simulink model "LLC_2converter"  (R2024a)
settings: Solver=ode1  StartTime=0.0  StopTime=0.05  FixedStep=1e-7  RelTol=1e-3
libraries: spsSeriesRLCBranchLib x6, spsCurrentMeasurementLib x4, spsDiodeLib x4, spsMosfetLib x2, spsVoltageMeasurementLib x2, spsLinearTransformerLib x1, spsPVArrayLib x1, sps_lib x1
settings Model: Creator=HP  LastModifiedBy=sampurnanand

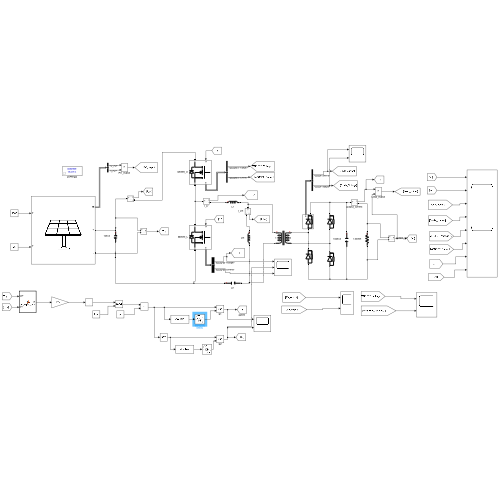
[thumbnail: Simulink's stored preview of the top-level diagram]
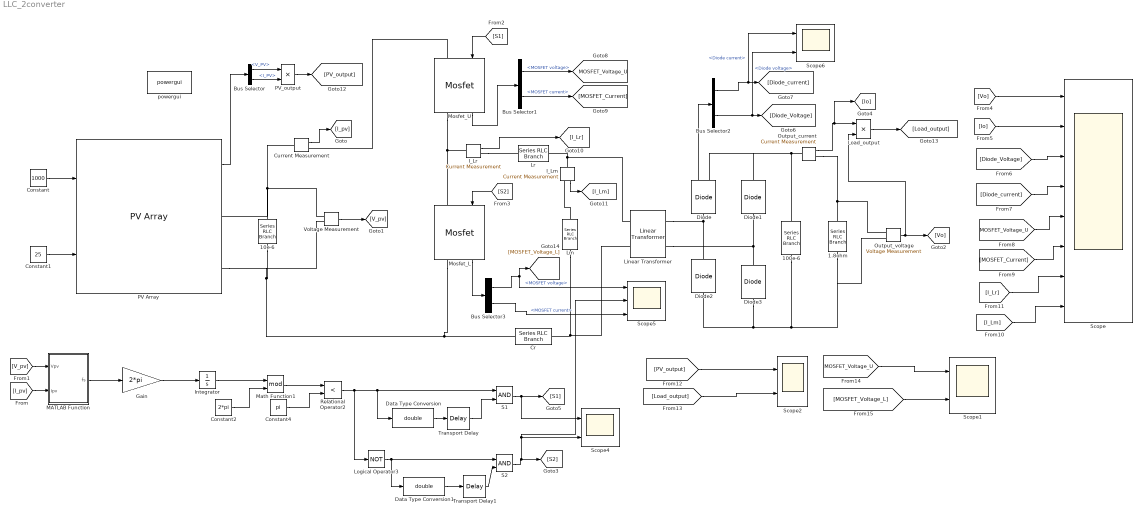
== system LLC_2converter ==
  1.8ohm : spsSeriesRLCBranchLib/Series RLC Branch  LConnTagsString=__new0  RConnTagsString=__new0  BranchType=R  Resistance=1.8  Inductance=1e-3  SetiL0=off  InitialCurrent=0  Capacitance=1e-6  Setx0=off  InitialVoltage=0  Measurements=None
  100e-6 : spsSeriesRLCBranchLib/Series RLC Branch  LConnTagsString=__new0  RConnTagsString=__new0  BranchType=C  Resistance=1  Inductance=1e-3  SetiL0=off  InitialCurrent=0  Capacitance=470e-6  Setx0=off  InitialVoltage=0  Measurements=None
  10e-6 : spsSeriesRLCBranchLib/Series RLC Branch  LConnTagsString=__new0  RConnTagsString=__new0  BranchType=C  Resistance=1  Inductance=1e-3  SetiL0=off  InitialCurrent=0  Capacitance=10e-5  Setx0=off  InitialVoltage=0  Measurements=None
  Bus Selector : BusSelector  OutputSignals=V_PV,I_PV
  Bus Selector1 : BusSelector  OutputSignals=MOSFET voltage,MOSFET current
  Bus Selector2 : BusSelector  OutputSignals=Diode current,Diode voltage
  Bus Selector3 : BusSelector  OutputSignals=MOSFET voltage,MOSFET current
  Constant : Constant  Value=1000
  Constant1 : Constant  Value=25
  Constant2 : Constant  Value=2*pi
  Constant4 : Constant  Value=pi
  Cr : spsSeriesRLCBranchLib/Series RLC Branch  LConnTagsString=__new0  RConnTagsString=__new0  BranchType=C  Resistance=1  Inductance=1e-3  SetiL0=off  InitialCurrent=0  Capacitance=3272e-9  Setx0=off  InitialVoltage=0  Measurements=None
  Current Measurement : spsCurrentMeasurementLib/Current Measurement  PhasorSimulation=off  OutputType=Complex  PSBequivalent=0
  Data Type Conversion : DataTypeConversion  OutDataTypeStr=double  SaturateOnIntegerOverflow=off  RndMeth=Floor
  Data Type Conversion1 : DataTypeConversion  OutDataTypeStr=double  SaturateOnIntegerOverflow=off  RndMeth=Floor
  Diode : spsDiodeLib/Diode  Ron=0.001  Lon=0  Vf=0.8  IC=0  UseSnubber=0  Rs=500  Cs=250e-9  Measurements=on
  Diode1 : spsDiodeLib/Diode  Ron=0.001  Lon=0  Vf=0.8  IC=0  UseSnubber=0  Rs=500  Cs=250e-9  Measurements=off
  Diode2 : spsDiodeLib/Diode  Ron=0.001  Lon=0  Vf=0.8  IC=0  UseSnubber=0  Rs=500  Cs=250e-9  Measurements=off
  Diode3 : spsDiodeLib/Diode  Ron=0.001  Lon=0  Vf=0.8  IC=0  UseSnubber=0  Rs=500  Cs=250e-9  Measurements=off
  Gain : Gain  Gain=2*pi
  I_Lm : spsCurrentMeasurementLib/Current Measurement  PhasorSimulation=off  OutputType=Complex  PSBequivalent=0
  I_Lr : spsCurrentMeasurementLib/Current Measurement  PhasorSimulation=off  OutputType=Complex  PSBequivalent=0
  Integrator : Integrator
  Linear Transformer : spsLinearTransformerLib/Linear Transformer  UNITS=SI  NominalPower=[2000 100e3]  winding1=[1 0 0]  winding2=[1 0 0]  ThreeWindings=off  winding3=[3.15e+05 0.7938 0.10107]  RmLm=[500 0]  Measurements=None  DataType=on
  Lm : spsSeriesRLCBranchLib/Series RLC Branch  LConnTagsString=__new0  RConnTagsString=__new0  BranchType=L  Resistance=1  Inductance=4e-6  SetiL0=off  InitialCurrent=0  Capacitance=1e-6  Setx0=off  InitialVoltage=0  Measurements=None
  Load_output : Product
  Logical Operator3 : Logic  Operator=NOT  AllPortsSameDT=off  OutDataTypeStr=boolean
  Lr : spsSeriesRLCBranchLib/Series RLC Branch  LConnTagsString=__new0  RConnTagsString=__new0  BranchType=L  Resistance=1  Inductance=0.77e-6  SetiL0=off  InitialCurrent=0  Capacitance=1e-6  Setx0=off  InitialVoltage=0  Measurements=None
  MATLAB Function : MATLAB Function  TreatAsAtomicUnit=on
  Math Function1 : Math  Operator=mod
  Mosfet_L : spsMosfetLib/Mosfet  Ron=0.01  Lon=0  Rd=0.01  Vfd=0  IC=0  Rs=1e5  Cs=inf  Measurements=on
  Mosfet_U : spsMosfetLib/Mosfet  Ron=0.01  Lon=0  Rd=0.01  Vfd=0  IC=0  Rs=1e5  Cs=inf  Measurements=on
  Output_current : spsCurrentMeasurementLib/Current Measurement  PhasorSimulation=off  OutputType=Complex  PSBequivalent=0
  Output_voltage : spsVoltageMeasurementLib/Voltage Measurement  PhasorSimulation=off  OutputType=Complex  PSBequivalent=0
  PV Array : spsPVArrayLib/PV Array  Npar=2  Nser=4  PlotType=array @ 25 deg.C & specified irradiances  S_vec="[ 1000  500  100 ]"  Temp_C_vec="[ 45 25  ]"  ModuleName=Andalay Solar TW-250-1-DC4-0-B  PlotWhenSelected=off  Pm=250.29  Ncell=72  Voc=36.8  Isc=8.75  Vm=30.9  Im=8.1  beta_Voc_pc=-0.36  alpha_Isc_pc=0.06  beta_Voc=-0.13248  alpha_Isc=0.00525  IL=8.7608  I0=2.9385e-10  nI=0.826  Rsh=125.9009  Rs=0.15507  RobustModel=off  RobustCellTemperature=313.3991  BAL=on  Tc=1e-6  Tfilter=5e-5
  PV_output : Product
  Relational Operator2 : RelationalOperator  Operator=<  OutDataTypeStr=boolean  RndMeth=Simplest  InputSameDT=off
  S1 : Logic  AllPortsSameDT=off  OutDataTypeStr=boolean
  S2 : Logic  AllPortsSameDT=off  OutDataTypeStr=boolean
  Scope : Scope  NumInputPorts=8
  Scope{1..2,4,6} (4 alike) : Scope  NumInputPorts=2
  Scope5 : Scope  NumInputPorts=3
  Transport Delay : TransportDelay  DelayTime=1e-6
  Transport Delay1 : TransportDelay  DelayTime=1e-6
  Voltage Measurement : spsVoltageMeasurementLib/Voltage Measurement  PhasorSimulation=off  OutputType=Complex  PSBequivalent=0
  powergui : sps_lib/powergui  Priority=1  SimulationMode=Discrete  SampleTime=1e-7  frequency=60  Iterations=50  frequencyindice=0  Pbase=100e6  ErrMax=1e-4  UnitsV=kV  UnitsW=MW  buscounter=0  FunctionMessages=off  echomessages=off  EnableUseOfTLC=off  CurrentSourceSwitches=off  DisableSnubberDevices=off  DisableRonSwitches=off  DisableVfSwitches=off  DisplayEquations=off  AutomaticDiscreteSolvers=off  SolverType=Tustin/Backward Euler (TBE)  Interpol=off  ExternalGateDelay=off  methode=off  Ts=100  x0status=blocks  SPID=on  SwTol=0  HookPort=off  NonlinearTolerance=1e-4  nMaxIteration=100  ContinueOnMaxIteration=off  RestoreLinks=warning  ResistiveCurrentMeasurement=off  Frange=[0:2:500]  Ylog=off  Xlog=on  ShowGrid=off  save=off  variable=ZData  structure=0  ZoomFFT=off  StartTime=0.0  cycles=1  DisplayStyle=1  fundamental=60  FreqAxis=off  MaxFrequency=1000  frequencyindicesteady=1  RmsSteady=1  display=off
  tag scope: MOSFET_Voltage_U=global
  wires:
  Data Type Conversion1/1 -> Transport Delay1/1
  Integrator/1 -> Math Function1/1
  Logical Operator3/1 -> S2/1, Data Type Conversion1/1
  [Diode_Voltage] -> Scope/3
  MATLAB Function/1(fs) -> Gain/1
  [Vo] -> Scope/1
  Load_output/1 -> [Load_output]
  Gain/1 -> Integrator/1
  Constant2/1 -> Math Function1/2
  [S1] -> Mosfet_U/1
  PV_output/1 -> [PV_output]
  Bus Selector/2 -> PV_output/2  "<I_PV>"
  [MOSFET_Current] -> Scope/6
  Math Function1/1 -> Relational Operator2/1
  Voltage Measurement/1 -> [V_pv]
  Output_current/1 -> [Io], Load_output/1
  Mosfet_U/1 -> Bus Selector1/1
  [S2] -> Mosfet_L/1
  I_Lr/1 -> [I_Lr]
  PV Array/1 -> Bus Selector/1
  Constant/1 -> PV Array/1
  [V_pv] -> MATLAB Function/1(Vpv)
  I_Lm/1 -> [I_Lm]
  [Diode_current] -> Scope/4
  Output_voltage/1 -> [Vo], Load_output/2
  Constant1/1 -> PV Array/2
  [MOSFET_Voltage_L] -> Scope1/2
  Bus Selector2/2 -> Scope6/2, [Diode_Voltage]  "<Diode voltage>"
  [PV_output] -> Scope2/1
  [MOSFET_Voltage_U] -> Scope1/1
  Diode/1 -> Bus Selector2/1
  Bus Selector3/1 -> Scope5/1, [MOSFET_Voltage_L]  "<MOSFET voltage>"
  [MOSFET_Voltage_U] -> Scope/5
  [Load_output] -> Scope2/2
  Bus Selector2/1 -> Scope6/1, [Diode_current]  "<Diode current>"
  [I_Lm] -> Scope/8
  Relational Operator2/1 -> Data Type Conversion/1, S1/1, Logical Operator3/1
  Current Measurement/1 -> [I_pv]
  Bus Selector/1 -> PV_output/1  "<V_PV>"
  Bus Selector1/1 -> [MOSFET_Voltage_U]  "<MOSFET voltage>"
  Bus Selector1/2 -> [MOSFET_Current]  "<MOSFET current>"
  [I_pv] -> MATLAB Function/2(Ipv)
  Transport Delay1/1 -> S2/2
  [Io] -> Scope/2
  Data Type Conversion/1 -> Transport Delay/1
  S1/1 -> Scope4/1, [S1]
  Constant4/1 -> Relational Operator2/2
  Transport Delay/1 -> S1/2
  Bus Selector3/2 -> Scope5/3  "<MOSFET current>"
  Mosfet_L/1 -> Bus Selector3/1
  [I_Lr] -> Scope/7
  S2/1 -> [S2], Scope5/2, Scope4/2
  connections:
  Output_current/LConn1 -- 100e-6/LConn1 -- Diode/RConn1 -- Diode1/RConn1
  1.8ohm/LConn1 -- Output_current/RConn1 -- Output_voltage/LConn1
  Cr/LConn1 -- Mosfet_L/RConn1 -- 10e-6/RConn1 -- Voltage Measurement/LConn2 -- PV Array/RConn2
  Voltage Measurement/LConn1 -- PV Array/RConn1 -- 10e-6/LConn1 -- Current Measurement/LConn1
  100e-6/RConn1 -- 1.8ohm/RConn1 -- Output_voltage/LConn2 -- Diode2/LConn1 -- Diode3/LConn1
  Linear Transformer/RConn2 -- Diode1/LConn1 -- Diode3/RConn1
  Linear Transformer/LConn2 -- Lm/RConn1 -- Cr/RConn1
  Linear Transformer/LConn1 -- I_Lm/LConn1 -- Lr/RConn1
  Linear Transformer/RConn1 -- Diode/LConn1 -- Diode2/RConn1
  Mosfet_L/LConn1 -- I_Lr/LConn1 -- Mosfet_U/RConn1
  Mosfet_U/LConn1 -- Current Measurement/RConn1
  Lm/LConn1 -- I_Lm/RConn1
  I_Lr/RConn1 -- Lr/LConn1

== matlab function LLC_2converter/MATLAB Function ==
  data: Vpv input; fs output; Ipv input
function fs = pv_mppt_pfm(Vpv, Ipv)
    % Persistent variables for memory across calls
    persistent Vold Pold Iold fs_prev timer P_filt V_filt I_filt;
    
    % Initialization on first call
    if isempty(Vold)
        Vold = 120;          % Nominal PV voltage baseline
        Pold = 0;            % Baseline power
        Iold = 0;            % Baseline current
        fs_prev = 100e3;     % Start at resonant frequency (100 kHz)
        timer = 0;
        P_filt = 0;
        V_filt = 120;
        I_filt = 0;
    end
    
    % Operational Limits & Parameters
    f_min = 60e3;        % Lower frequency bound (60 kHz)
    f_max = 120e3;       % Upper frequency bound (120 kHz)
    L = 0.5;             % Step scaling factor
    Ts = 1e-7;           % Simulation step size
    T_mppt = 2e-3;       % MPPT execution interval (2 ms)
    
    % Instantaneous Power
    Ppv = Vpv * Ipv;
    
    % Low-pass filter to eliminate high-frequency ripple
    alpha = 0.05;
    P_filt = alpha * Ppv + (1 - alpha) * P_filt;
    V_filt = alpha * Vpv + (1 - alpha) * V_filt;
    I_filt = alpha * Ipv + (1 - alpha) * I_filt;
    
    % Increment timer
    timer = timer + Ts;
    
    % Execute MPPT every T_mppt
    if timer >= T_mppt
        timer = 0;
        
        dP = P_filt - Pold;
        dV = V_filt - Vold;
        dI = I_filt - Iold;
        
        % Adaptive step size M
        M = L * abs(dP + dV * dI);
        M_min = 10;   
        M_max = 500; % Reduced max step size for finer convergence
        M = min(max(M, M_min), M_max);
        
        % Correct PFM logic for LLC:
        % dP > 0 and dV > 0 -> We moved right on P-V curve -> Decrease fs to extract more power
        if abs(dP) > 0.1
            if dP > 0
                if dV > 0
                    fs_prev = fs_prev - M; % Move toward Vmpp
                else
                    fs_prev = fs_prev + M;
                end
            else
                if dV > 0
                    fs_prev = fs_prev + M;
                else
                    fs_prev = fs_prev - M;
                end
            end
        end
        
        % Update states
        Vold = V_filt;
        Pold = P_filt;
        Iold = I_filt;
    end
    
    % Bound frequency around resonance
    if fs_prev > f_max
        fs_prev = f_max;
    elseif fs_prev < f_min
        fs_prev = f_min;
    end
    
    fs = fs_prev;
end
